simulink model "LGS_allFaultsDeselected"  (R2019b)
settings: Solver=FixedStepDiscrete  StartTime=0.0  StopTime=45.0  FixedStep=0.1  RelTol=1e-3
model workspace (MAT data in the model file):
  fipData : object (value not decoded)
  fipName : object (value not decoded)
  stepSize = 0.1
libraries: LibFaultInjectionControls x190, commrandsrc3 x70, simulink x3, LibFailureCondition x1
(part 2 of 41)

== system LGS_allFaultsDeselected/Analogical switch and general electro-valve and pressure sensor/General EV ==
  note: [true, false]
  In1 : Inport
  In2 : Inport  Port=2
  General EV FIP : Subsystem  Commented=on  mask(FailureInjectionPoint){}
      mask help: FailureInjectionPoint
      mask init: same as LGS_allFaultsDeselected/Analogical switch and general electro-valve and pressure sensor/Analogical switch/Analog Switch FIP
      settings: OpenFcn=|
      | open_system(gcb,'mask');
      | 
      | treeValues = FailureInjectionPointHelper.getAllFmAndParamsAsTreeString(gcb);
      | mo = Simulink.Mask.get(gcb);
      | dc = mo.getDialogControl('GbFmInfo');
      | treeView = dc.getDialogControl('TreeViewFM');
      | treeView.TreeItems = {};
      | treeView.TreeItems = treeValues;
      mask Help: FailureInjectionPoint
      mask DialogControl Control7 Prompt: Containing Failure Modes
      mask DialogControl BtnMoveUp Prompt: Move up
      mask DialogControl BtnMoveUp Callback:
      | %Get name of the failure mode block
      | mo = Simulink.Mask.get(gcb);
      | dc = mo.getDialogControl('GbFmInfo');
      | treeView = dc.getDialogControl('TreeViewFM');
      | try
      |     a = treeView.getSelectedItems();
      |     p = split(a, '/'); %name of failure mode block is p{1}
      | catch
      |     return;
      | end
      | 
      | %Save port handles
      | lh = get_param([gcb,'/',p{1}],'LineHandles');
      | ph = get_param([gcb,'/',p{1}],'PortHandles');
      | this_in = ph.Inport(1);
      | this_out = ph.Outport(1);
      | 
      | last_block = get_param(lh.Inport(1),'SrcBlockHandle');
      | last_block_type = get_param(last_block,'BlockType');
      | if strcmp(last_block_type,'Inport')
      |     return;
      | end
      | lb_lh = get_param(last_block,'LineHandles');
      | 
      | last_out = get_param(lh.Inport(1),'SrcPortHandle');
      | last_in = get_param(lb_lh.Inport(1),'DstPortHandle');
      | next_to_last_out = get_param(lb_lh.Inport(1),'SrcPortHandle');
      | next_in = get_param(lh.Outport(1),'DstPortHandle');
      | 
      | %Delete connecting lines
      | delete_line(lh.Inport(1));
      | delete_line(lh.Outport(1));
      | delete_line(lb_lh.Inport(1));
      | 
      | % Generate new lines
      | add_line(gcb, last_out, next_in, 'autorouting', 'smart');
      | add_line(gcb, this_out, last_in, 'autorouting', 'smart');
      | add_line(gcb, next_to_last_out, this_in, 'autorouting', 'smart');
      | 
      | %Rearrange system
      | Simulink.BlockDiagram.arrangeSystem(gcb);
      | 
      | %Refresh
      | treeValues = FailureInjectionPointHelper.getAllFmAndParamsAsTreeString(gcb);
      | mo = Simulink.Mask.get(gcb);
      | dc = mo.getDialogControl('GbFmInfo');
      | treeView = dc.getDialogControl('TreeViewFM');
      | treeView.TreeItems = {};
      | treeView.TreeItems = treeValues;
      mask DialogControl BtnMoveDown Prompt: Move down
      mask DialogControl BtnMoveDown Callback:
      | %Get name of the failure mode block
      | mo = Simulink.Mask.get(gcb);
      | dc = mo.getDialogControl('GbFmInfo');
      | treeView = dc.getDialogControl('TreeViewFM');
      | try
      |     a = treeView.getSelectedItems();
      |     p = split(a, '/'); %name of failure mode block is p{1}
      | catch
      |     return;
      | end
      | 
      | %Save port handles
      | lh = get_param([gcb,'/',p{1}],'LineHandles');
      | ph = get_param([gcb,'/',p{1}],'PortHandles');
      | this_in = ph.Inport(1);
      | this_out = ph.Outport(1);
      | 
      | next_block = get_param(lh.Outport(1),'DstBlockHandle');
      | next_block_type = get_param(next_block,'BlockType');
      | if strcmp(next_block_type,'Outport')
      |     return;
      | end
      | nb_lh = get_param(next_block,'LineHandles');
      | 
      | last_out = get_param(lh.Inport(1),'SrcPortHandle');
      | next_out = get_param(nb_lh.Outport(1),'SrcPortHandle');
      | next_but_one_in = get_param(nb_lh.Outport(1),'DstPortHandle');
      | next_in = get_param(lh.Outport(1),'DstPortHandle');
      | 
      | %Delete connecting lines
      | delete_line(lh.Inport(1));
      | delete_line(lh.Outport(1));
      | delete_line(nb_lh.Outport(1));
      | 
      | % Generate new lines
      | add_line(gcb, last_out, next_in, 'autorouting', 'smart');
      | add_line(gcb, next_out, this_in, 'autorouting', 'smart');
      | add_line(gcb, this_out, next_but_one_in, 'autorouting', 'smart');
      | 
      | %Rearrange system
      | Simulink.BlockDiagram.arrangeSystem(gcb);
      | 
      | %Refresh
      | treeValues = FailureInjectionPointHelper.getAllFmAndParamsAsTreeString(gcb);
      | mo = Simulink.Mask.get(gcb);
      | dc = mo.getDialogControl('GbFmInfo');
      | treeView = dc.getDialogControl('TreeViewFM');
      | treeView.TreeItems = {};
      | treeView.TreeItems = treeValues;
      mask DialogControl TreeViewFM Prompt: Failure Mode Information
      mask DialogControl BtnOpen Prompt: Open FIP
      mask DialogControl BtnOpen Callback: open_system(gcb,'force');
      mask DialogControl BtnNew Prompt: New
      mask DialogControl BtnNew Callback:
      | dialog_fipManager_single(gcb, '');
      | 
      | %Enable move, edit, delete buttons
      | mo = Simulink.Mask.get(gcb);
      | mo.getDialogControl('BtnMoveUp').Enabled = 'on';
      | mo.getDialogControl('BtnMoveDown').Enabled = 'on';
      | mo.getDialogControl('BtnEdit').Enabled = 'on';
      | mo.getDialogControl('BtnDelete').Enabled = 'on';
      mask DialogControl BtnEdit Prompt: Edit
      mask DialogControl BtnEdit Callback:
      | mo = Simulink.Mask.get(gcb);
      | dc = mo.getDialogControl('GbFmInfo');
      | treeView = dc.getDialogControl('TreeViewFM');
      | try
      |     a = treeView.getSelectedItems();
      |     p = split(a, '/');
      | catch
      |     return;
      | end
      | dialog_fipManager_single(gcb, p{1});
      mask DialogControl BtnDelete Prompt: Delete
      mask DialogControl BtnDelete Callback:
      | %Get name of the failure mode block
      | mo = Simulink.Mask.get(gcb);
      | dc = mo.getDialogControl('GbFmInfo');
      | treeView = dc.getDialogControl('TreeViewFM');
      | try
      |     a = treeView.getSelectedItems();
      |     p = split(a, '/'); %name of failure mode block is p{1}
      | catch
      |     return;
      | end
      | 
      | %Save outport handle of the last and inport handle of the next block
      | lh = get_param([gcb,'/',p{1}],'LineHandles');
      | last_out = get_param(lh.Inport(1),'SrcPortHandle');
      | next_in = get_param(lh.Outport(1),'DstPortHandle');
      | 
      | %Delete connecting lines and failure mode block
      | delete_line(lh.Inport(1));
      | delete_line(lh.Outport(1));
      | fm_handle = get_param([gcb,'/',p{1}],'Handle');
      | delete_block(fm_handle);
      | 
      | % Generate new line from outport last to inport next
      | add_line(gcb, last_out, next_in, 'autorouting', 'smart');
      | 
      | %Rearrange system
      | Simulink.BlockDiagram.arrangeSystem(gcb);
      | 
      | %Disable move, edit, delete buttons in case all FMs are deleted
      | last_block = get_param(last_out,'Parent');
      | last_is_inport = strcmp(get_param(last_block,'BlockType'),'Inport');
      | next_block = get_param(next_in,'Parent');
      | next_is_outport = strcmp(get_param(next_block,'BlockType'),'Outport');
      | if (last_is_inport && next_is_outport)
      |     mo.getDialogControl('BtnMoveUp').Enabled = 'off';
      |     mo.getDialogControl('BtnMoveDown').Enabled = 'off';
      |     mo.getDialogControl('BtnEdit').Enabled = 'off';
      |     mo.getDialogControl('BtnDelete').Enabled = 'off';
      | end
      | 
      | %Refresh
      | treeValues = FailureInjectionPointHelper.getAllFmAndParamsAsTreeString(gcb);
      | mo = Simulink.Mask.get(gcb);
      | dc = mo.getDialogControl('GbFmInfo');
      | treeView = dc.getDialogControl('TreeViewFM');
      | treeView.TreeItems = {};
      | treeView.TreeItems = treeValues;
      mask DialogControl BtnRefresh Prompt: Refresh
      mask DialogControl BtnRefresh Callback:
      | set_param(gcb,'LinkStatus','none');
      | 
      | treeValues = FailureInjectionPointHelper.getAllFmAndParamsAsTreeString(gcb);
      | mo = Simulink.Mask.get(gcb);
      | dc = mo.getDialogControl('GbFmInfo');
      | treeView = dc.getDialogControl('TreeViewFM');
      | treeView.TreeItems = {};
      | treeView.TreeItems = treeValues;
      mask Display: image('icons/failure_injection_point.png','center')
  Trigger FIP : LibFaultInjectionControls/Trigger FIP  Active=off  MaintenanceTask=1  RiskTime=1  FailureRate=1.0E-3  isDSF=off  DSFjson=JSON
      settings: SourceProductName=Fault Injection Controls
  general EV : Stateflow chart  TreatAsAtomicUnit=on
  Out1 : Outport
  wires:
  In1/1 -> general EV/1(generalEVPresure_in)
  In2/1 -> general EV/2(signal_in)
  general EV/1(generalEVPresure_out) -> Out1/1
  Trigger FIP/1 -> general EV/3(fail)

== system LGS_allFaultsDeselected/Analogical switch and general electro-valve and pressure sensor/sensor switch closed ==
  note: [true, false]
  note: [true, false]
  note: [true, false]
  sensor input : Inport  OutDataTypeStr=boolean
  Bus Creator3 : BusCreator  Inputs=3
  FIP1 : Subsystem
  FIP2 : Subsystem
  FIP3 : Subsystem
  sensor output : Outport
  wires:
  FIP2/1(Out1) -> Bus Creator3/2  "signal2"
  FIP1/1(Out1) -> Bus Creator3/1  "signal1"
  FIP3/1(Out1) -> Bus Creator3/3  "signal3"
  sensor input/1 -> FIP3/1(In1), FIP2/1(In1), FIP1/1(In1)
  Bus Creator3/1 -> sensor output/1

== system LGS_allFaultsDeselected/Analogical switch and general electro-valve and pressure sensor/sensor system pressurized ==
  note: [true, false]
  note: [true, false]
  note: [true, false]
  sensor input : Inport  OutDataTypeStr=boolean
  Bus Creator3 : BusCreator  Inputs=3
  FIP1 : Subsystem
  FIP2 : Subsystem
  FIP3 : Subsystem
  sensor output : Outport
  wires:
  FIP2/1(Out1) -> Bus Creator3/2  "signal2"
  FIP1/1(Out1) -> Bus Creator3/1  "signal1"
  FIP3/1(Out1) -> Bus Creator3/3  "signal3"
  sensor input/1 -> FIP3/1(In1), FIP2/1(In1), FIP1/1(In1)
  Bus Creator3/1 -> sensor output/1

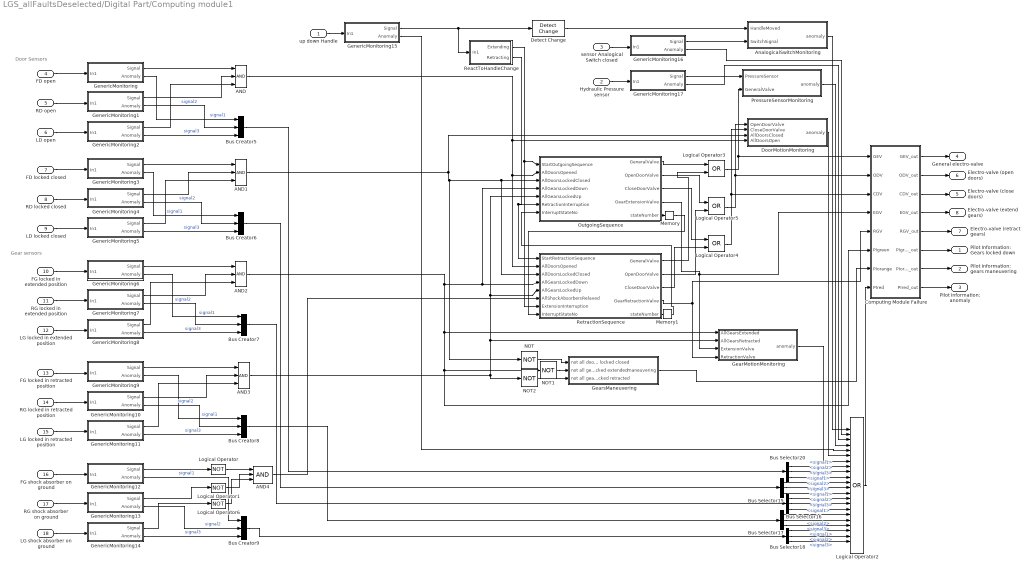
== system LGS_allFaultsDeselected/Digital Part/Computing module1 ==
  note: Gear sensors
  note: Door Sensors
  up down Handle : Inport
  Hydraulic Pressure sensor : Inport  Port=2
  " sensor Analogical Switch closed" : Inport  Port=3
  FD open : Inport  Port=4
  RD open : Inport  Port=5
  LD open : Inport  Port=6
  FD locked closed : Inport  Port=7
  RD locked closed : Inport  Port=8
  LD locked closed : Inport  Port=9
  FG locked in extended position : Inport  Port=10
  RG locked in extended position : Inport  Port=11
  LG locked in extended position : Inport  Port=12
  FG locked in retracted position : Inport  Port=13
  RG locked in retracted position : Inport  Port=14
  LG locked in retracted position : Inport  Port=15
  FG shock absorber on ground : Inport  Port=16
  RG shock absorber on ground : Inport  Port=17
  LG shock absorber on ground : Inport  Port=18
  AND{,1..4} (5 alike) : Logic  Inputs=3  IconShape=distinctive  AllPortsSameDT=off  OutDataTypeStr=boolean
  AnalogicalSwitchMonitoring : Stateflow chart  TreatAsAtomicUnit=on
  Bus Creator{5..9} (5 alike) : BusCreator  Inputs=3
  Bus Selector{15..18,20} (5 alike) : BusSelector  OutputSignals=signal1,signal2,signal3
  Computing Module Failure : Subsystem
  Detect Change : simulink/Logic and Bit Operations/Detect Change  vinit=1  OutDataTypeStr=boolean
  DoorMotionMonitoring : Stateflow chart  TreatAsAtomicUnit=on
  GearMotionMonitoring : Stateflow chart  TreatAsAtomicUnit=on
  GearsManeuvering : Subsystem
  GenericMonitoring : Subsystem
  GenericMonitoring1 : Subsystem
  GenericMonitoring10 : Subsystem
  GenericMonitoring11 : Subsystem
  GenericMonitoring12 : Subsystem
  GenericMonitoring13 : Subsystem
  GenericMonitoring14 : Subsystem
  GenericMonitoring15 : Subsystem
  GenericMonitoring16 : Subsystem
  GenericMonitoring17 : Subsystem
  GenericMonitoring2 : Subsystem
  GenericMonitoring3 : Subsystem
  GenericMonitoring4 : Subsystem
  GenericMonitoring5 : Subsystem
  GenericMonitoring6 : Subsystem
  GenericMonitoring7 : Subsystem
  GenericMonitoring8 : Subsystem
  GenericMonitoring9 : Subsystem
  Logical Operator : Logic  Operator=NOT  AllPortsSameDT=off  OutDataTypeStr=boolean
  Logical Operator1 : Logic  Operator=NOT  AllPortsSameDT=off  OutDataTypeStr=boolean
  Logical Operator2 : Logic  Operator=OR  Inputs=22  AllPortsSameDT=off  OutDataTypeStr=boolean
  Logical Operator3 : Logic  Operator=OR  AllPortsSameDT=off  OutDataTypeStr=boolean
  Logical Operator4 : Logic  Operator=OR  AllPortsSameDT=off  OutDataTypeStr=boolean
  Logical Operator5 : Logic  Operator=OR  AllPortsSameDT=off  OutDataTypeStr=boolean
  Logical Operator6 : Logic  Operator=NOT  AllPortsSameDT=off  OutDataTypeStr=boolean
  Memory : Memory  InheritSampleTime=on
  Memory1 : Memory  InheritSampleTime=on
  NOT : Logic  Operator=NOT  IconShape=distinctive  AllPortsSameDT=off  OutDataTypeStr=boolean
  NOT1 : Logic  Operator=NOT  IconShape=distinctive  AllPortsSameDT=off  OutDataTypeStr=boolean
  NOT2 : Logic  Operator=NOT  IconShape=distinctive  AllPortsSameDT=off  OutDataTypeStr=boolean
  OutgoingSequence : Stateflow chart  TreatAsAtomicUnit=on
  PressureSensorMonitoring : Stateflow chart  TreatAsAtomicUnit=on
  ReactToHandleChange : Subsystem
  RetractionSequence : Stateflow chart  TreatAsAtomicUnit=on
  Pilot Information: Gears locked down : Outport  OutDataTypeStr=boolean
  Pilot Information: gears maneuvering : Outport  Port=2  OutDataTypeStr=boolean
  Pilot Information: anomaly : Outport  Port=3  OutDataTypeStr=boolean
  General electro-valve : Outport  Port=4
  Electro-valve (close doors) : Outport  Port=5
  Electro-valve (open doors) : Outport  Port=6
  Electro-valve (retract gears) : Outport  Port=7
  Electro-valve (extend gears) : Outport  Port=8
  wires:
  ReactToHandleChange/1(Extending) -> RetractionSequence/7(ExtensionInterruption), OutgoingSequence/1(StartOutgoingSequence)
  OutgoingSequence/1(GeneralValve) -> Logical Operator3/1
  OutgoingSequence/2(OpenDoorValve) -> Logical Operator5/1
  OutgoingSequence/4(GearExtensionValve) -> GearMotionMonitoring/3(ExtensionValve), Computing Module Failure/4(EGV)
  OutgoingSequence/3(CloseDoorValve) -> Logical Operator4/1
  AND/1 -> DoorMotionMonitoring/4(AllDoorsOpen), RetractionSequence/2(AllDoorsOpened), OutgoingSequence/2(AllDoorsOpened)
  AND1/1 -> NOT/1, RetractionSequence/3(AllDoorsLockedClosed), OutgoingSequence/3(AllDoorsLockedClosed), DoorMotionMonitoring/3(AllDoorsClosed)
  AND2/1 -> GearMotionMonitoring/1(AllGearsExtended), NOT1/1, Computing Module Failure/6(PIgreen), RetractionSequence/4(AllGearsLockedDown), OutgoingSequence/4(AllGearsLockedDown)
  GearsManeuvering/1(maneuvering) -> Computing Module Failure/7(PIorange)
  AnalogicalSwitchMonitoring/1(anomaly) -> Logical Operator2/1
  Detect Change/1 -> AnalogicalSwitchMonitoring/1(HandleMoved)
  " sensor Analogical Switch closed"/1 -> GenericMonitoring16/1(In1)
  Hydraulic Pressure sensor/1 -> GenericMonitoring17/1(In1)
  PressureSensorMonitoring/1(anomaly) -> Logical Operator2/4
  DoorMotionMonitoring/1(anomaly) -> Logical Operator2/6
  GearMotionMonitoring/1(anomaly) -> Logical Operator2/7
  Logical Operator2/1 -> Computing Module Failure/8(PIred)
  RetractionSequence/1(GeneralValve) -> Logical Operator3/2
  Logical Operator3/1 -> PressureSensorMonitoring/2(GeneralValve), Computing Module Failure/1(GEV)
  RetractionSequence/3(CloseDoorValve) -> Logical Operator4/2
  Logical Operator4/1 -> DoorMotionMonitoring/2(CloseDoorValve), Computing Module Failure/3(CDV)
  RetractionSequence/2(OpenDoorValve) -> Logical Operator5/2
  Logical Operator5/1 -> DoorMotionMonitoring/1(OpenDoorValve), Computing Module Failure/2(ODV)
  RetractionSequence/4(GearRetractionValve) -> GearMotionMonitoring/4(RetractionValve), Computing Module Failure/5(RGV)
  Bus Creator5/1 -> Bus Selector20/1
  AND3/1 -> NOT2/1, GearMotionMonitoring/2(AllGearsRetracted), RetractionSequence/5(AllGearsLockedUp), OutgoingSequence/5(AllGearsLockedUp)
  ReactToHandleChange/2(Retracting) -> RetractionSequence/1(StartRetractionSequence), OutgoingSequence/6(RetractionInterruption)
  Bus Selector15/1 -> Logical Operator2/11  "<signal1>"
  Bus Selector15/2 -> Logical Operator2/12  "<signal2>"
  Bus Selector15/3 -> Logical Operator2/13  "<signal3>"
  Bus Selector16/1 -> Logical Operator2/14  "<signal1>"
  Bus Selector16/2 -> Logical Operator2/15  "<signal2>"
  Bus Selector16/3 -> Logical Operator2/16  "<signal3>"
  Bus Selector17/1 -> Logical Operator2/17  "<signal1>"
  Bus Selector17/2 -> Logical Operator2/18  "<signal2>"
  Bus Selector17/3 -> Logical Operator2/19  "<signal3>"
  Bus Selector18/1 -> Logical Operator2/20  "<signal1>"
  Bus Selector18/2 -> Logical Operator2/21  "<signal2>"
  Bus Selector18/3 -> Logical Operator2/22  "<signal3>"
  Bus Selector20/1 -> Logical Operator2/8  "<signal1>"
  Bus Selector20/2 -> Logical Operator2/9  "<signal2>"
  Bus Selector20/3 -> Logical Operator2/10  "<signal3>"
  Bus Creator6/1 -> Bus Selector15/1
  Bus Creator7/1 -> Bus Selector16/1
  Bus Creator8/1 -> Bus Selector17/1
  Bus Creator9/1 -> Bus Selector18/1
  GenericMonitoring17/1(Signal) -> PressureSensorMonitoring/1(PressureSensor)
  GenericMonitoring16/1(Signal) -> AnalogicalSwitchMonitoring/2(SwitchSignal)
  GenericMonitoring16/2(Anomaly) -> Logical Operator2/2
  up down Handle/1 -> GenericMonitoring15/1(In1)
  GenericMonitoring15/2(Anomaly) -> Logical Operator2/5
  GenericMonitoring17/2(Anomaly) -> Logical Operator2/3
  Memory/1 -> RetractionSequence/8(InterruptStateNo)
  Memory1/1 -> OutgoingSequence/7(InterruptStateNo)
  OutgoingSequence/5(stateNumber) -> Memory/1
  RetractionSequence/5(stateNumber) -> Memory1/1
  Computing Module Failure/1(GEV_out) -> General electro-valve/1
  Computing Module Failure/2(ODV_out) -> Electro-valve (open doors)/1
  Computing Module Failure/3(CDV_out) -> Electro-valve (close doors)/1
  Computing Module Failure/4(EGV_out) -> Electro-valve (extend gears)/1
  Computing Module Failure/5(RGV_out) -> Electro-valve (retract gears)/1
  Computing Module Failure/6(PIgreen_out) -> Pilot Information: Gears locked down/1
  Computing Module Failure/7(PIorange_out) -> Pilot Information: gears maneuvering/1
  Computing Module Failure/8(PIred_out) -> Pilot Information: anomaly/1
  AND4/1 -> RetractionSequence/6(AllShockAbsorbersRelaxed)
  GenericMonitoring15/1(Signal) -> Detect Change/1, ReactToHandleChange/1(In1)
  NOT/1 -> GearsManeuvering/1(not all doors locked closed)
  NOT1/1 -> GearsManeuvering/2(not all gears locked extended)
  NOT2/1 -> GearsManeuvering/3(not all gears locked retracted)
  GenericMonitoring7/1(Signal) -> AND2/2
  GenericMonitoring8/1(Signal) -> AND2/3
  GenericMonitoring6/1(Signal) -> AND2/1
  GenericMonitoring10/2(Anomaly) -> Bus Creator8/2  "signal2"
  GenericMonitoring5/1(Signal) -> AND1/3
  GenericMonitoring6/2(Anomaly) -> Bus Creator7/1  "signal1"
  Logical Operator6/1 -> AND4/3
  LG shock absorber on ground/1 -> GenericMonitoring14/1(In1)
  GenericMonitoring10/1(Signal) -> AND3/2
  GenericMonitoring11/1(Signal) -> AND3/3
  RD open/1 -> GenericMonitoring1/1(In1)
  GenericMonitoring4/1(Signal) -> AND1/2
  GenericMonitoring12/2(Anomaly) -> Bus Creator9/1  "signal1"
  GenericMonitoring7/2(Anomaly) -> Bus Creator7/2  "signal2"
  GenericMonitoring14/2(Anomaly) -> Bus Creator9/3  "signal3"
  GenericMonitoring/1(Signal) -> AND/1
  Logical Operator/1 -> AND4/1
  GenericMonitoring/2(Anomaly) -> Bus Creator5/1  "signal1"
  GenericMonitoring4/2(Anomaly) -> Bus Creator6/2  "signal2"
  GenericMonitoring14/1(Signal) -> Logical Operator6/1
  GenericMonitoring12/1(Signal) -> Logical Operator/1
  GenericMonitoring11/2(Anomaly) -> Bus Creator8/3  "signal3"
  RG locked in extended position/1 -> GenericMonitoring7/1(In1)
  GenericMonitoring9/1(Signal) -> AND3/1
  RG shock absorber on ground/1 -> GenericMonitoring13/1(In1)
  GenericMonitoring2/1(Signal) -> AND/3
  GenericMonitoring1/2(Anomaly) -> Bus Creator5/2  "signal2"
  GenericMonitoring3/2(Anomaly) -> Bus Creator6/1  "signal1"
  FG shock absorber on ground/1 -> GenericMonitoring12/1(In1)
  RG locked in retracted position/1 -> GenericMonitoring10/1(In1)
  GenericMonitoring2/2(Anomaly) -> Bus Creator5/3  "signal3"
  GenericMonitoring3/1(Signal) -> AND1/1
  LG locked in retracted position/1 -> GenericMonitoring11/1(In1)
  Logical Operator1/1 -> AND4/2
  GenericMonitoring13/2(Anomaly) -> Bus Creator9/2  "signal2"
  LD locked closed/1 -> GenericMonitoring5/1(In1)
  GenericMonitoring13/1(Signal) -> Logical Operator1/1
  GenericMonitoring5/2(Anomaly) -> Bus Creator6/3  "signal3"
  FD locked closed/1 -> GenericMonitoring3/1(In1)
  FG locked in extended position/1 -> GenericMonitoring6/1(In1)
  GenericMonitoring1/1(Signal) -> AND/2
  GenericMonitoring9/2(Anomaly) -> Bus Creator8/1  "signal1"
  FG locked in retracted position/1 -> GenericMonitoring9/1(In1)
  RD locked closed/1 -> GenericMonitoring4/1(In1)
  FD open/1 -> GenericMonitoring/1(In1)
  LD open/1 -> GenericMonitoring2/1(In1)
  GenericMonitoring8/2(Anomaly) -> Bus Creator7/3  "signal3"
  LG locked in extended position/1 -> GenericMonitoring8/1(In1)

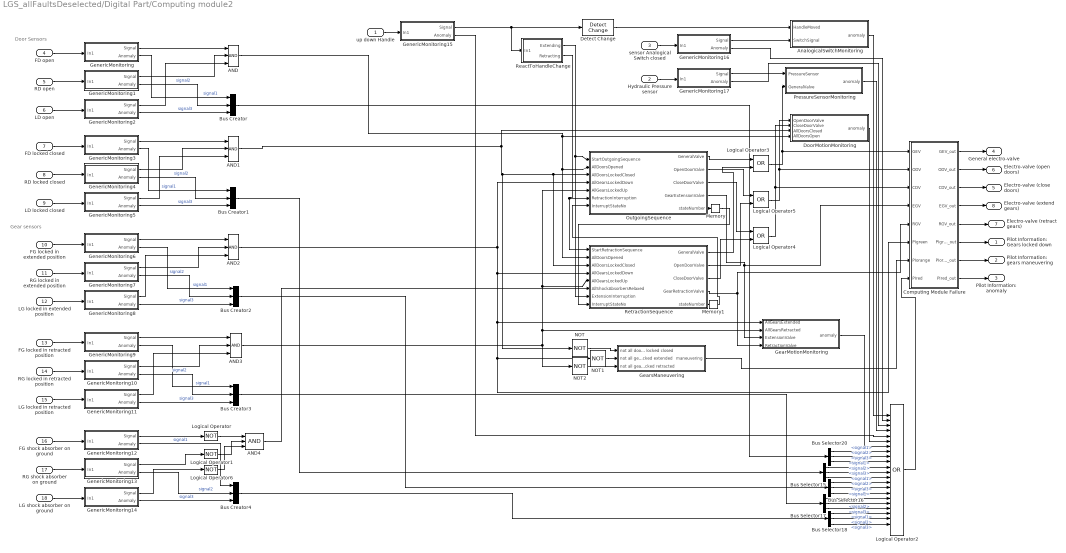
== system LGS_allFaultsDeselected/Digital Part/Computing module2 ==
  note: Gear sensors
  note: Door Sensors
  up down Handle : Inport
  Hydraulic Pressure sensor : Inport  Port=2
  " sensor Analogical Switch closed" : Inport  Port=3
  FD open : Inport  Port=4
  RD open : Inport  Port=5
  LD open : Inport  Port=6
  FD locked closed : Inport  Port=7
  RD locked closed : Inport  Port=8
  LD locked closed : Inport  Port=9
  FG locked in extended position : Inport  Port=10
  RG locked in extended position : Inport  Port=11
  LG locked in extended position : Inport  Port=12
  FG locked in retracted position : Inport  Port=13
  RG locked in retracted position : Inport  Port=14
  LG locked in retracted position : Inport  Port=15
  FG shock absorber on ground : Inport  Port=16
  RG shock absorber on ground : Inport  Port=17
  LG shock absorber on ground : Inport  Port=18
  AND{,1..4} (5 alike) : Logic  Inputs=3  IconShape=distinctive  AllPortsSameDT=off  OutDataTypeStr=boolean
  AnalogicalSwitchMonitoring : Stateflow chart  TreatAsAtomicUnit=on
  Bus Creator{,1..4} (5 alike) : BusCreator  Inputs=3
  Bus Selector{15..18,20} (5 alike) : BusSelector  OutputSignals=signal1,signal2,signal3
  Computing Module Failure : Subsystem
  Detect Change : simulink/Logic and Bit Operations/Detect Change  vinit=1  OutDataTypeStr=boolean
  DoorMotionMonitoring : Stateflow chart  TreatAsAtomicUnit=on
  GearMotionMonitoring : Stateflow chart  TreatAsAtomicUnit=on
  GearsManeuvering : Subsystem
  GenericMonitoring : Subsystem
  GenericMonitoring1 : Subsystem
  GenericMonitoring10 : Subsystem
  GenericMonitoring11 : Subsystem
  GenericMonitoring12 : Subsystem
  GenericMonitoring13 : Subsystem
  GenericMonitoring14 : Subsystem
  GenericMonitoring15 : Subsystem
  GenericMonitoring16 : Subsystem
  GenericMonitoring17 : Subsystem
  GenericMonitoring2 : Subsystem
  GenericMonitoring3 : Subsystem
  GenericMonitoring4 : Subsystem
  GenericMonitoring5 : Subsystem
  GenericMonitoring6 : Subsystem
  GenericMonitoring7 : Subsystem
  GenericMonitoring8 : Subsystem
  GenericMonitoring9 : Subsystem
  Logical Operator : Logic  Operator=NOT  AllPortsSameDT=off  OutDataTypeStr=boolean
  Logical Operator1 : Logic  Operator=NOT  AllPortsSameDT=off  OutDataTypeStr=boolean
  Logical Operator2 : Logic  Operator=OR  Inputs=22  AllPortsSameDT=off  OutDataTypeStr=boolean
  Logical Operator3 : Logic  Operator=OR  AllPortsSameDT=off  OutDataTypeStr=boolean
  Logical Operator4 : Logic  Operator=OR  AllPortsSameDT=off  OutDataTypeStr=boolean
  Logical Operator5 : Logic  Operator=OR  AllPortsSameDT=off  OutDataTypeStr=boolean
  Logical Operator6 : Logic  Operator=NOT  AllPortsSameDT=off  OutDataTypeStr=boolean
  Memory : Memory  InheritSampleTime=on
  Memory1 : Memory  InheritSampleTime=on
  NOT : Logic  Operator=NOT  IconShape=distinctive  AllPortsSameDT=off  OutDataTypeStr=boolean
  NOT1 : Logic  Operator=NOT  IconShape=distinctive  AllPortsSameDT=off  OutDataTypeStr=boolean
  NOT2 : Logic  Operator=NOT  IconShape=distinctive  AllPortsSameDT=off  OutDataTypeStr=boolean
  OutgoingSequence : Stateflow chart  TreatAsAtomicUnit=on
  PressureSensorMonitoring : Stateflow chart  TreatAsAtomicUnit=on
  ReactToHandleChange : Subsystem
  RetractionSequence : Stateflow chart  TreatAsAtomicUnit=on
  Pilot Information: Gears locked down : Outport  OutDataTypeStr=boolean
  Pilot Information: gears maneuvering : Outport  Port=2  OutDataTypeStr=boolean
  Pilot Information: anomaly : Outport  Port=3  OutDataTypeStr=boolean
  General electro-valve : Outport  Port=4
  Electro-valve (close doors) : Outport  Port=5
  Electro-valve (open doors) : Outport  Port=6
  Electro-valve (retract gears) : Outport  Port=7
  Electro-valve (extend gears) : Outport  Port=8
  wires:
  ReactToHandleChange/1(Extending) -> RetractionSequence/7(ExtensionInterruption), OutgoingSequence/1(StartOutgoingSequence)
  OutgoingSequence/1(GeneralValve) -> Logical Operator3/1
  OutgoingSequence/2(OpenDoorValve) -> Logical Operator5/1
  OutgoingSequence/4(GearExtensionValve) -> Computing Module Failure/4(EGV), GearMotionMonitoring/3(ExtensionValve)
  OutgoingSequence/3(CloseDoorValve) -> Logical Operator4/1
  FD open/1 -> GenericMonitoring/1(In1)
  RD open/1 -> GenericMonitoring1/1(In1)
  LD open/1 -> GenericMonitoring2/1(In1)
  AND/1 -> DoorMotionMonitoring/4(AllDoorsOpen), RetractionSequence/2(AllDoorsOpened), OutgoingSequence/2(AllDoorsOpened)
  FD locked closed/1 -> GenericMonitoring3/1(In1)
  RD locked closed/1 -> GenericMonitoring4/1(In1)
  LD locked closed/1 -> GenericMonitoring5/1(In1)
  AND1/1 -> NOT/1, RetractionSequence/3(AllDoorsLockedClosed), OutgoingSequence/3(AllDoorsLockedClosed), DoorMotionMonitoring/3(AllDoorsClosed)
  FG locked in extended position/1 -> GenericMonitoring6/1(In1)
  RG locked in extended position/1 -> GenericMonitoring7/1(In1)
  LG locked in extended position/1 -> GenericMonitoring8/1(In1)
  FG locked in retracted position/1 -> GenericMonitoring9/1(In1)
  RG locked in retracted position/1 -> GenericMonitoring10/1(In1)
  LG locked in retracted position/1 -> GenericMonitoring11/1(In1)
  LG shock absorber on ground/1 -> GenericMonitoring14/1(In1)
  AND2/1 -> Computing Module Failure/6(PIgreen), NOT1/1, GearMotionMonitoring/1(AllGearsExtended), RetractionSequence/4(AllGearsLockedDown), OutgoingSequence/4(AllGearsLockedDown)
  GearsManeuvering/1(maneuvering) -> Computing Module Failure/7(PIorange)
  FG shock absorber on ground/1 -> GenericMonitoring12/1(In1)
  GenericMonitoring12/1(Signal) -> Logical Operator/1
  GenericMonitoring13/1(Signal) -> Logical Operator1/1
  GenericMonitoring14/1(Signal) -> Logical Operator6/1
  AnalogicalSwitchMonitoring/1(anomaly) -> Logical Operator2/1
  Detect Change/1 -> AnalogicalSwitchMonitoring/1(HandleMoved)
  " sensor Analogical Switch closed"/1 -> GenericMonitoring16/1(In1)
  Hydraulic Pressure sensor/1 -> GenericMonitoring17/1(In1)
  PressureSensorMonitoring/1(anomaly) -> Logical Operator2/4
  DoorMotionMonitoring/1(anomaly) -> Logical Operator2/6
  GearMotionMonitoring/1(anomaly) -> Logical Operator2/7
  Logical Operator2/1 -> Computing Module Failure/8(PIred)
  RG shock absorber on ground/1 -> GenericMonitoring13/1(In1)
  RetractionSequence/1(GeneralValve) -> Logical Operator3/2
  Logical Operator3/1 -> Computing Module Failure/1(GEV), PressureSensorMonitoring/2(GeneralValve)
  RetractionSequence/3(CloseDoorValve) -> Logical Operator4/2
  Logical Operator4/1 -> Computing Module Failure/3(CDV), DoorMotionMonitoring/2(CloseDoorValve)
  RetractionSequence/2(OpenDoorValve) -> Logical Operator5/2
  Logical Operator5/1 -> Computing Module Failure/2(ODV), DoorMotionMonitoring/1(OpenDoorValve)
  RetractionSequence/4(GearRetractionValve) -> Computing Module Failure/5(RGV), GearMotionMonitoring/4(RetractionValve)
  GenericMonitoring/2(Anomaly) -> Bus Creator/1  "signal1"
  GenericMonitoring2/2(Anomaly) -> Bus Creator/3  "signal3"
  GenericMonitoring1/2(Anomaly) -> Bus Creator/2  "signal2"
  Bus Creator/1 -> Bus Selector20/1
  AND3/1 -> GearMotionMonitoring/2(AllGearsRetracted), RetractionSequence/5(AllGearsLockedUp), OutgoingSequence/5(AllGearsLockedUp), NOT2/1
  ReactToHandleChange/2(Retracting) -> RetractionSequence/1(StartRetractionSequence), OutgoingSequence/6(RetractionInterruption)
  Bus Selector15/1 -> Logical Operator2/11  "<signal1>"
  Bus Selector15/2 -> Logical Operator2/12  "<signal2>"
  Bus Selector15/3 -> Logical Operator2/13  "<signal3>"
  Bus Selector16/1 -> Logical Operator2/14  "<signal1>"
  Bus Selector16/2 -> Logical Operator2/15  "<signal2>"
  Bus Selector16/3 -> Logical Operator2/16  "<signal3>"
  Bus Selector17/1 -> Logical Operator2/17  "<signal1>"
  Bus Selector17/2 -> Logical Operator2/18  "<signal2>"
  Bus Selector17/3 -> Logical Operator2/19  "<signal3>"
  Bus Selector18/1 -> Logical Operator2/20  "<signal1>"
  Bus Selector18/2 -> Logical Operator2/21  "<signal2>"
  Bus Selector18/3 -> Logical Operator2/22  "<signal3>"
  Bus Selector20/1 -> Logical Operator2/8  "<signal1>"
  Bus Selector20/2 -> Logical Operator2/9  "<signal2>"
  Bus Selector20/3 -> Logical Operator2/10  "<signal3>"
  GenericMonitoring12/2(Anomaly) -> Bus Creator4/1  "signal1"
  GenericMonitoring3/2(Anomaly) -> Bus Creator1/1  "signal1"
  GenericMonitoring4/2(Anomaly) -> Bus Creator1/2  "signal2"
  GenericMonitoring5/2(Anomaly) -> Bus Creator1/3  "signal3"
  Bus Creator1/1 -> Bus Selector15/1
  GenericMonitoring8/2(Anomaly) -> Bus Creator2/3  "signal3"
  GenericMonitoring6/2(Anomaly) -> Bus Creator2/1  "signal1"
  GenericMonitoring7/2(Anomaly) -> Bus Creator2/2  "signal2"
  Bus Creator2/1 -> Bus Selector16/1
  GenericMonitoring11/2(Anomaly) -> Bus Creator3/3  "signal3"
  GenericMonitoring10/2(Anomaly) -> Bus Creator3/2  "signal2"
  GenericMonitoring9/2(Anomaly) -> Bus Creator3/1  "signal1"
  Bus Creator3/1 -> Bus Selector17/1
  GenericMonitoring13/2(Anomaly) -> Bus Creator4/2  "signal2"
  GenericMonitoring14/2(Anomaly) -> Bus Creator4/3  "signal3"
  Bus Creator4/1 -> Bus Selector18/1
  Logical Operator/1 -> AND4/1
  Logical Operator6/1 -> AND4/3
  GenericMonitoring17/1(Signal) -> PressureSensorMonitoring/1(PressureSensor)
  GenericMonitoring16/1(Signal) -> AnalogicalSwitchMonitoring/2(SwitchSignal)
  GenericMonitoring16/2(Anomaly) -> Logical Operator2/2
  up down Handle/1 -> GenericMonitoring15/1(In1)
  GenericMonitoring15/2(Anomaly) -> Logical Operator2/5
  GenericMonitoring17/2(Anomaly) -> Logical Operator2/3
  Memory/1 -> RetractionSequence/8(InterruptStateNo)
  Memory1/1 -> OutgoingSequence/7(InterruptStateNo)
  OutgoingSequence/5(stateNumber) -> Memory/1
  RetractionSequence/5(stateNumber) -> Memory1/1
  Computing Module Failure/1(GEV_out) -> General electro-valve/1
  Computing Module Failure/2(ODV_out) -> Electro-valve (open doors)/1
  Computing Module Failure/3(CDV_out) -> Electro-valve (close doors)/1
  Computing Module Failure/4(EGV_out) -> Electro-valve (extend gears)/1
  Computing Module Failure/5(RGV_out) -> Electro-valve (retract gears)/1
  Computing Module Failure/6(PIgreen_out) -> Pilot Information: Gears locked down/1
  Computing Module Failure/7(PIorange_out) -> Pilot Information: gears maneuvering/1
  Computing Module Failure/8(PIred_out) -> Pilot Information: anomaly/1
  AND4/1 -> RetractionSequence/6(AllShockAbsorbersRelaxed)
  GenericMonitoring15/1(Signal) -> Detect Change/1, ReactToHandleChange/1(In1)
  GenericMonitoring/1(Signal) -> AND/1
  GenericMonitoring1/1(Signal) -> AND/2
  GenericMonitoring2/1(Signal) -> AND/3
  GenericMonitoring3/1(Signal) -> AND1/1
  GenericMonitoring4/1(Signal) -> AND1/2
  GenericMonitoring5/1(Signal) -> AND1/3
  GenericMonitoring6/1(Signal) -> AND2/1
  GenericMonitoring7/1(Signal) -> AND2/2
  GenericMonitoring8/1(Signal) -> AND2/3
  GenericMonitoring9/1(Signal) -> AND3/1
  GenericMonitoring10/1(Signal) -> AND3/2
  GenericMonitoring11/1(Signal) -> AND3/3
  NOT/1 -> GearsManeuvering/1(not all doors locked closed)
  NOT1/1 -> GearsManeuvering/2(not all gears locked extended)
  NOT2/1 -> GearsManeuvering/3(not all gears locked retracted)
  Logical Operator1/1 -> AND4/2

== system LGS_allFaultsDeselected/Doors/EV close doors ==
  In1 : Inport
  In2 : Inport  Port=2
  EV close doors : Stateflow chart  TreatAsAtomicUnit=on
  EV close doors FIP : Subsystem  Commented=on  mask(FailureInjectionPoint){}
      mask help: FailureInjectionPoint
      mask init: same as LGS_allFaultsDeselected/Analogical switch and general electro-valve and pressure sensor/Analogical switch/Analog Switch FIP
      settings: OpenFcn=|
      | open_system(gcb,'mask');
      | 
      | treeValues = FailureInjectionPointHelper.getAllFmAndParamsAsTreeString(gcb);
      | mo = Simulink.Mask.get(gcb);
      | dc = mo.getDialogControl('GbFmInfo');
      | treeView = dc.getDialogControl('TreeViewFM');
      | treeView.TreeItems = {};
      | treeView.TreeItems = treeValues;
      mask Help: FailureInjectionPoint
      mask DialogControl Control7 Prompt: Containing Failure Modes
      mask DialogControl BtnMoveUp Prompt: Move up
      mask DialogControl BtnMoveUp Callback:
      | %Get name of the failure mode block
      | mo = Simulink.Mask.get(gcb);
      | dc = mo.getDialogControl('GbFmInfo');
      | treeView = dc.getDialogControl('TreeViewFM');
      | try
      |     a = treeView.getSelectedItems();
      |     p = split(a, '/'); %name of failure mode block is p{1}
      | catch
      |     return;
      | end
      | 
      | %Save port handles
      | lh = get_param([gcb,'/',p{1}],'LineHandles');
      | ph = get_param([gcb,'/',p{1}],'PortHandles');
      | this_in = ph.Inport(1);
      | this_out = ph.Outport(1);
      | 
      | last_block = get_param(lh.Inport(1),'SrcBlockHandle');
      | last_block_type = get_param(last_block,'BlockType');
      | if strcmp(last_block_type,'Inport')
      |     return;
      | end
      | lb_lh = get_param(last_block,'LineHandles');
      | 
      | last_out = get_param(lh.Inport(1),'SrcPortHandle');
      | last_in = get_param(lb_lh.Inport(1),'DstPortHandle');
      | next_to_last_out = get_param(lb_lh.Inport(1),'SrcPortHandle');
      | next_in = get_param(lh.Outport(1),'DstPortHandle');
      | 
      | %Delete connecting lines
      | delete_line(lh.Inport(1));
      | delete_line(lh.Outport(1));
      | delete_line(lb_lh.Inport(1));
      | 
      | % Generate new lines
      | add_line(gcb, last_out, next_in, 'autorouting', 'smart');
      | add_line(gcb, this_out, last_in, 'autorouting', 'smart');
      | add_line(gcb, next_to_last_out, this_in, 'autorouting', 'smart');
      | 
      | %Rearrange system
      | Simulink.BlockDiagram.arrangeSystem(gcb);
      | 
      | %Refresh
      | treeValues = FailureInjectionPointHelper.getAllFmAndParamsAsTreeString(gcb);
      | mo = Simulink.Mask.get(gcb);
      | dc = mo.getDialogControl('GbFmInfo');
      | treeView = dc.getDialogControl('TreeViewFM');
      | treeView.TreeItems = {};
      | treeView.TreeItems = treeValues;
      mask DialogControl BtnMoveDown Prompt: Move down
      mask DialogControl BtnMoveDown Callback:
      | %Get name of the failure mode block
      | mo = Simulink.Mask.get(gcb);
      | dc = mo.getDialogControl('GbFmInfo');
      | treeView = dc.getDialogControl('TreeViewFM');
      | try
      |     a = treeView.getSelectedItems();
      |     p = split(a, '/'); %name of failure mode block is p{1}
      | catch
      |     return;
      | end
      | 
      | %Save port handles
      | lh = get_param([gcb,'/',p{1}],'LineHandles');
      | ph = get_param([gcb,'/',p{1}],'PortHandles');
      | this_in = ph.Inport(1);
      | this_out = ph.Outport(1);
      | 
      | next_block = get_param(lh.Outport(1),'DstBlockHandle');
      | next_block_type = get_param(next_block,'BlockType');
      | if strcmp(next_block_type,'Outport')
      |     return;
      | end
      | nb_lh = get_param(next_block,'LineHandles');
      | 
      | last_out = get_param(lh.Inport(1),'SrcPortHandle');
      | next_out = get_param(nb_lh.Outport(1),'SrcPortHandle');
      | next_but_one_in = get_param(nb_lh.Outport(1),'DstPortHandle');
      | next_in = get_param(lh.Outport(1),'DstPortHandle');
      | 
      | %Delete connecting lines
      | delete_line(lh.Inport(1));
      | delete_line(lh.Outport(1));
      | delete_line(nb_lh.Outport(1));
      | 
      | % Generate new lines
      | add_line(gcb, last_out, next_in, 'autorouting', 'smart');
      | add_line(gcb, next_out, this_in, 'autorouting', 'smart');
      | add_line(gcb, this_out, next_but_one_in, 'autorouting', 'smart');
      | 
      | %Rearrange system
      | Simulink.BlockDiagram.arrangeSystem(gcb);
      | 
      | %Refresh
      | treeValues = FailureInjectionPointHelper.getAllFmAndParamsAsTreeString(gcb);
      | mo = Simulink.Mask.get(gcb);
      | dc = mo.getDialogControl('GbFmInfo');
      | treeView = dc.getDialogControl('TreeViewFM');
      | treeView.TreeItems = {};
      | treeView.TreeItems = treeValues;
      mask DialogControl TreeViewFM Prompt: Failure Mode Information
      mask DialogControl BtnOpen Prompt: Open FIP
      mask DialogControl BtnOpen Callback: open_system(gcb,'force');
      mask DialogControl BtnNew Prompt: New
      mask DialogControl BtnNew Callback:
      | dialog_fipManager_single(gcb, '');
      | 
      | %Enable move, edit, delete buttons
      | mo = Simulink.Mask.get(gcb);
      | mo.getDialogControl('BtnMoveUp').Enabled = 'on';
      | mo.getDialogControl('BtnMoveDown').Enabled = 'on';
      | mo.getDialogControl('BtnEdit').Enabled = 'on';
      | mo.getDialogControl('BtnDelete').Enabled = 'on';
      mask DialogControl BtnEdit Prompt: Edit
      mask DialogControl BtnEdit Callback:
      | mo = Simulink.Mask.get(gcb);
      | dc = mo.getDialogControl('GbFmInfo');
      | treeView = dc.getDialogControl('TreeViewFM');
      | try
      |     a = treeView.getSelectedItems();
      |     p = split(a, '/');
      | catch
      |     return;
      | end
      | dialog_fipManager_single(gcb, p{1});
      mask DialogControl BtnDelete Prompt: Delete
      mask DialogControl BtnDelete Callback:
      | %Get name of the failure mode block
      | mo = Simulink.Mask.get(gcb);
      | dc = mo.getDialogControl('GbFmInfo');
      | treeView = dc.getDialogControl('TreeViewFM');
      | try
      |     a = treeView.getSelectedItems();
      |     p = split(a, '/'); %name of failure mode block is p{1}
      | catch
      |     return;
      | end
      | 
      | %Save outport handle of the last and inport handle of the next block
      | lh = get_param([gcb,'/',p{1}],'LineHandles');
      | last_out = get_param(lh.Inport(1),'SrcPortHandle');
      | next_in = get_param(lh.Outport(1),'DstPortHandle');
      | 
      | %Delete connecting lines and failure mode block
      | delete_line(lh.Inport(1));
      | delete_line(lh.Outport(1));
      | fm_handle = get_param([gcb,'/',p{1}],'Handle');
      | delete_block(fm_handle);
      | 
      | % Generate new line from outport last to inport next
      | add_line(gcb, last_out, next_in, 'autorouting', 'smart');
      | 
      | %Rearrange system
      | Simulink.BlockDiagram.arrangeSystem(gcb);
      | 
      | %Disable move, edit, delete buttons in case all FMs are deleted
      | last_block = get_param(last_out,'Parent');
      | last_is_inport = strcmp(get_param(last_block,'BlockType'),'Inport');
      | next_block = get_param(next_in,'Parent');
      | next_is_outport = strcmp(get_param(next_block,'BlockType'),'Outport');
      | if (last_is_inport && next_is_outport)
      |     mo.getDialogControl('BtnMoveUp').Enabled = 'off';
      |     mo.getDialogControl('BtnMoveDown').Enabled = 'off';
      |     mo.getDialogControl('BtnEdit').Enabled = 'off';
      |     mo.getDialogControl('BtnDelete').Enabled = 'off';
      | end
      | 
      | %Refresh
      | treeValues = FailureInjectionPointHelper.getAllFmAndParamsAsTreeString(gcb);
      | mo = Simulink.Mask.get(gcb);
      | dc = mo.getDialogControl('GbFmInfo');
      | treeView = dc.getDialogControl('TreeViewFM');
      | treeView.TreeItems = {};
      | treeView.TreeItems = treeValues;
      mask DialogControl BtnRefresh Prompt: Refresh
      mask DialogControl BtnRefresh Callback:
      | set_param(gcb,'LinkStatus','none');
      | 
      | treeValues = FailureInjectionPointHelper.getAllFmAndParamsAsTreeString(gcb);
      | mo = Simulink.Mask.get(gcb);
      | dc = mo.getDialogControl('GbFmInfo');
      | treeView = dc.getDialogControl('TreeViewFM');
      | treeView.TreeItems = {};
      | treeView.TreeItems = treeValues;
      mask Display: image('icons/failure_injection_point.png','center')
  Memory : Memory  InheritSampleTime=on
  Trigger FIP : LibFaultInjectionControls/Trigger FIP  Active=off  MaintenanceTask=1  RiskTime=1  FailureRate=1.0E-3  isDSF=off  DSFjson=JSON
      settings: SourceProductName=Fault Injection Controls
  Out1 : Outport
  wires:
  Memory/1 -> EV close doors/1(signal_in)
  In1/1 -> Memory/1
  In2/1 -> EV close doors/2(EVCloseDoorsPresure_in)
  EV close doors/1(EVCloseDoorsPresure_out) -> Out1/1
  Trigger FIP/1 -> EV close doors/3(fail)
